simulink model "SMC_Thermal"  (R2024a)
settings: Solver=ode4  StartTime=0.0  StopTime=0.5  RelTol=1e-3
values from neighbouring files (symbols this model uses):
  C = 100e-6    (= 0.0001)    [converter_parameter.m]
  r_load = 5    [converter_parameter.m]
  V_fc = 14.4    [converter_parameter.m]
undefined symbols (not defined in the file or in its folder): plecs
libraries: eePwmGenerator x2
settings Model: Creator=qaromose  LastModifiedBy=QUDUS
settings DebuggingCC: UnconnectedInputMsg=warning  UnconnectedOutputMsg=warning  UnconnectedLineMsg=warning
settings ModelReferenceCC: EnableRefExpFcnMdlSchedulingChecks=on
settings RTWCC: GPUComputeCapability=3.5  DLArmComputeVersion=19.05

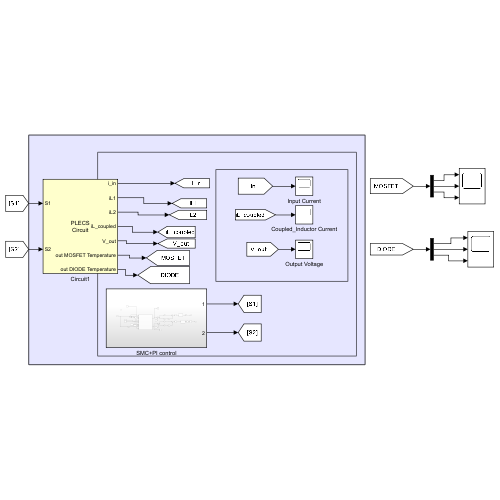
[thumbnail: Simulink's stored preview of the top-level diagram]
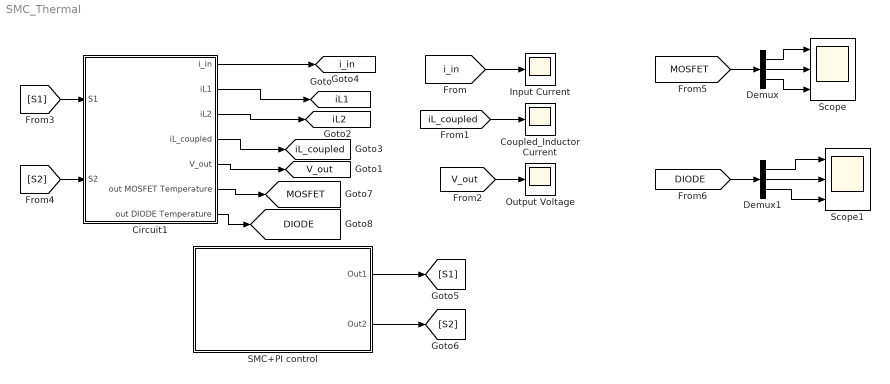
== system SMC_Thermal ==
  Circuit1 : Subsystem  LoadFcn=plecs('sl', 200);  InitFcn=plecs('sl', 214);  StartFcn=plecs('sl', 208);  StopFcn=plecs('sl', 209);  mask(PlecsCircuit){PLECSData=<binary blob, 16104 chars, not shown>}
      mask prompts: PLECSData "PLECS Data (Do not delete or modify!)"
      mask init:
      | % PLACE CUSTOM INITIALIZATIONS ABOVE
      | % DO NOT REMOVE
      | plecs('sl', 215);
      | % DO NOT REMOVE
      settings: CopyFcn=plecs('sl', 203);  DeleteFcn=plecs('sl', 205);  UndoDeleteFcn=plecs('sl', 206);  PreSaveFcn=plecs('sl', 211);  PostSaveFcn=plecs('sl', 201);  NameChangeFcn=plecs('sl', 210);  DestroyFcn=plecs('sl', 207);  PreCopyFcn=plecs('sl', 216);  OpenFcn=plecs('sl', 202);  ErrorFcn=plerrorfcn
      mask Help: eval('plecs(''help'', ''qthelp:///creatingacircuit.html'')')
      mask Display: disp('PLECS\nCircuit')
  Coupled_Inductor Current : Scope
  Demux : Demux  Outputs=3
  Demux1 : Demux  Outputs=3
  Input Current : Scope
  Output Voltage : Scope
  SMC+PI control : Subsystem
  Scope : Scope  NumInputPorts=3
  Scope1 : Scope  NumInputPorts=3
  tag scope: DIODE=global, MOSFET=global, V_out=global, iL1=global, iL2=global, iL_coupled=global, i_in=global
  wires:
  SMC+PI control/2(Out2) -> [S2]
  [V_out] -> Output Voltage/1
  SMC+PI control/1(Out1) -> [S1]
  [iL_coupled] -> Coupled_Inductor Current/1
  [i_in] -> Input Current/1
  [S1] -> Circuit1/1(S1)
  [S2] -> Circuit1/2(S2)
  Circuit1/1(i_in) -> [i_in]
  Circuit1/2(iL1) -> [iL1]
  Circuit1/3(iL2) -> [iL2]
  Circuit1/4(iL_coupled) -> [iL_coupled]
  Circuit1/5(V_out) -> [V_out]
  Circuit1/6(out MOSFET Temperature) -> [MOSFET]
  Circuit1/7(out DIODE Temperature) -> [DIODE]
  [MOSFET] -> Demux/1
  [DIODE] -> Demux1/1
  Demux/1 -> Scope/1
  Demux/2 -> Scope/2
  Demux/3 -> Scope/3
  Demux1/2 -> Scope1/2
  Demux1/3 -> Scope1/3
  Demux1/1 -> Scope1/1

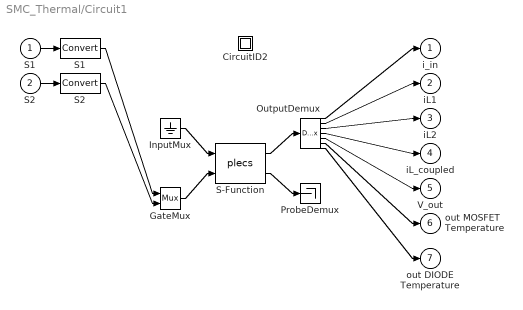
== system SMC_Thermal/Circuit1 ==
  S1 : Inport  PortDimensions=1
  S2 : Inport  Port=2  PortDimensions=1
  " CircuitID2 " : Subsystem
  " GateMux " : Mux  Inputs=[ 1 1 ]
  " InputMux " : Ground
  " OutputDemux " : Demux  Outputs=[ 1 1 1 2 1 3 3 ]
  " ProbeDemux " : Terminator
  " S-Function " : S-Function  FunctionName=plecs  SFunctionDeploymentMode=off  EnableBusSupport=off
  " S1 " : DataTypeConversion
  " S2 " : DataTypeConversion
  i_in : Outport  PortDimensions=1
  iL1 : Outport  Port=2  PortDimensions=1
  iL2 : Outport  Port=3  PortDimensions=1
  iL_coupled : Outport  Port=4  PortDimensions=2
  V_out : Outport  Port=5  PortDimensions=1
  out MOSFET Temperature : Outport  Port=6  PortDimensions=3
  out DIODE Temperature : Outport  Port=7  PortDimensions=3
  wires:
  " InputMux "/1 -> " S-Function "/1
  " GateMux "/1 -> " S-Function "/2
  " S-Function "/1 -> " OutputDemux "/1
  " S-Function "/2 -> " ProbeDemux "/1
  S1/1 -> " S1 "/1
  " S1 "/1 -> " GateMux "/1
  S2/1 -> " S2 "/1
  " S2 "/1 -> " GateMux "/2
  " OutputDemux "/1 -> i_in/1
  " OutputDemux "/2 -> iL1/1
  " OutputDemux "/3 -> iL2/1
  " OutputDemux "/4 -> iL_coupled/1
  " OutputDemux "/5 -> V_out/1
  " OutputDemux "/6 -> out MOSFET Temperature/1
  " OutputDemux "/7 -> out DIODE Temperature/1

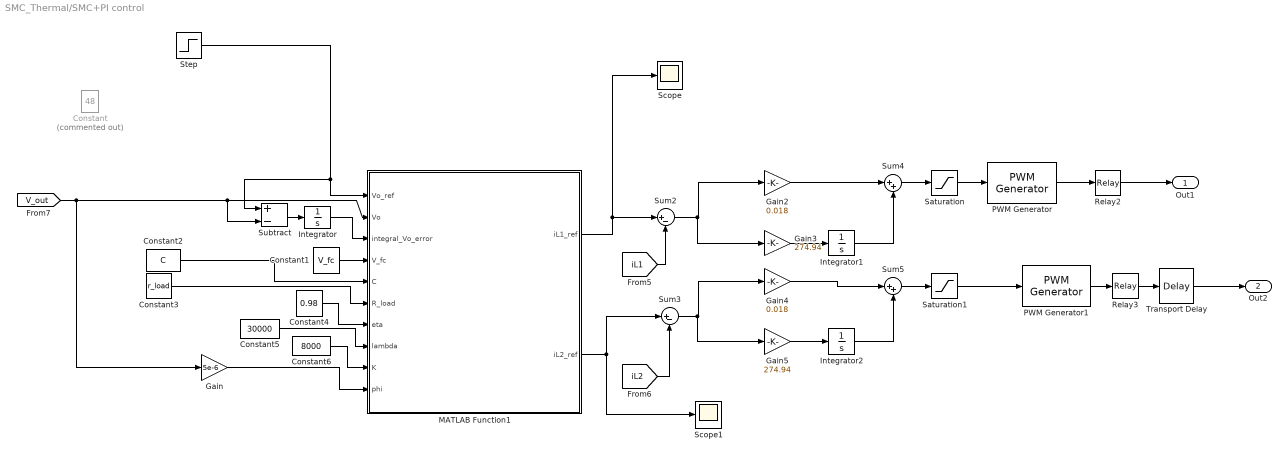
== system SMC_Thermal/SMC+PI control ==
  Constant : Constant  Commented=on  Value=48
  Constant1 : Constant  Value=V_fc
  Constant2 : Constant  Value=C
  Constant3 : Constant  Value=r_load
  Constant4 : Constant  Value=0.98
  Constant5 : Constant  Value=30000
  Constant6 : Constant  Value=8000
  Gain : Gain  Gain=5e-6
  Gain2 : Gain  Gain=0.018
  Gain3 : Gain  Gain=274.94
  Gain4 : Gain  Gain=0.018
  Gain5 : Gain  Gain=274.94
  Integrator : Integrator
  Integrator1 : Integrator
  Integrator2 : Integrator
  MATLAB Function1 : MATLAB Function  TreatAsAtomicUnit=on
  PWM Generator : eePwmGenerator/PWM Generator  CarrCount=Up  Tper=2e-5  Tdelay=0  Ts=0
  PWM Generator1 : eePwmGenerator/PWM Generator  CarrCount=Up  Tper=2e-5  Tdelay=0  Ts=0
  Relay2 : Relay
  Relay3 : Relay
  Saturation : Saturate  UpperLimit=0.97  LowerLimit=0.1
  Saturation1 : Saturate  UpperLimit=0.97  LowerLimit=0.1
  Scope : Scope
  Scope1 : Scope
  Step : Step  Time=0.2  Before=48  After=40  SampleTime=0
  Subtract : Sum  Inputs=+-
  Sum2 : Sum  Inputs=|+-
  Sum3 : Sum  Inputs=|+-
  Sum4 : Sum  Inputs=|++
  Sum5 : Sum  Inputs=|++
  Transport Delay : TransportDelay  DelayTime=1e-5
  Out1 : Outport
  Out2 : Outport  Port=2
  wires:
  Relay2/1 -> Out1/1
  Relay3/1 -> Transport Delay/1
  Sum2/1 -> Gain3/1, Gain2/1
  [V_out] -> Gain/1, Subtract/2, MATLAB Function1/2(Vo)
  Saturation/1 -> PWM Generator/1
  [iL1] -> Sum2/2
  Subtract/1 -> Integrator/1
  Transport Delay/1 -> Out2/1
  Sum3/1 -> Gain5/1, Gain4/1
  MATLAB Function1/1(iL1_ref) -> Scope/1, Sum2/1
  MATLAB Function1/2(iL2_ref) -> Sum3/1, Scope1/1
  PWM Generator/1 -> Relay2/1
  Gain4/1 -> Sum5/1
  Sum4/1 -> Saturation/1
  Gain5/1 -> Integrator2/1
  Integrator2/1 -> Sum5/2
  Gain3/1 -> Integrator1/1
  PWM Generator1/1 -> Relay3/1
  Integrator1/1 -> Sum4/2
  Integrator/1 -> MATLAB Function1/3(integral_Vo_error)
  Gain2/1 -> Sum4/1
  Saturation1/1 -> PWM Generator1/1
  Sum5/1 -> Saturation1/1
  [iL2] -> Sum3/2
  Constant2/1 -> MATLAB Function1/5(C)
  Constant3/1 -> MATLAB Function1/6(R_load)
  Constant4/1 -> MATLAB Function1/7(eta)
  Constant5/1 -> MATLAB Function1/8(lambda)
  Constant6/1 -> MATLAB Function1/9(K)
  Gain/1 -> MATLAB Function1/10(phi)
  Constant1/1 -> MATLAB Function1/4(V_fc)
  Step/1 -> Subtract/1, MATLAB Function1/1(Vo_ref)

== system SMC_Thermal/Circuit1/ CircuitID2  ==

== matlab function SMC_Thermal/SMC+PI control/MATLAB Function1 ==
  data: Vo_ref input; Vo input; integral_Vo_error input; iL1_ref output; iL2_ref output; V_fc input; C input; R_load input; eta input; lambda input; K input; phi input
function [iL1_ref, iL2_ref] = Outer_SMC(Vo_ref, Vo, integral_Vo_error, V_fc, C, R_load, eta, lambda, K, phi)
    %% System Parameters (Optimized for ±0.5V Error)
%     V_fc = 14.4;          % Input voltage [V] (measured under load)
%     C = 100e-6;          % Output capacitance [F] 
%     R_load = 5;          % Load resistance [Ω] (48V/500W = 4.608Ω, adjust if needed)
%     eta = 0.97;          % desired efficiency (compensate for losses at higher Vo)
%     lambda = 2500;       % Aggressive integral gain (eliminate steady-state error)
%     K = 600;             % High robustness gain (dominate uncertainties)
%     phi = 0.5 * Vo_ref;% Adaptive boundary layer (0.5% of Vo_ref)
    
    %% Voltage error (Vo_ref - Vo)
    e_V = Vo_ref - Vo;
    
    %% Sliding surface
    S = e_V + lambda * integral_Vo_error;
    
    %% Adaptive boundary layer saturation
    if abs(S) <= phi
        sat_term = S / phi;   % Linear region
    else
        sat_term = sign(S);   % Reaching mode
    end
    
    %% Feedforward term (with efficiency compensation)
    iL_ref_eq = (Vo_ref^2) / (V_fc * R_load * eta);  % Critical adjustment
    
    %% Feedback term (scaled for precision)
    robustness_term = (C / V_fc) * (lambda * e_V + K * sat_term); 
    
    %% Total current reference (remove clamp or set hardware-safe limit)
    iL_ref_total = iL_ref_eq + robustness_term;
    % iL_ref_total = max(min(iL_ref_total, 100), 0);  % Example: 100A limit
    
    %% Split equally for 2-phase IBC
    iL1_ref = iL_ref_total / 2;  
    iL2_ref = iL_ref_total / 2;
end
